simulink model "Energy_Cost03_04_2012"  (Simulink 7.5)
settings: Solver=ode45  StartTime=0.0  StopTime=24  RelTol=1e-3
model workspace: external: MAT-File (data not in the file)
libraries: simulink x4
(part 2 of 2)

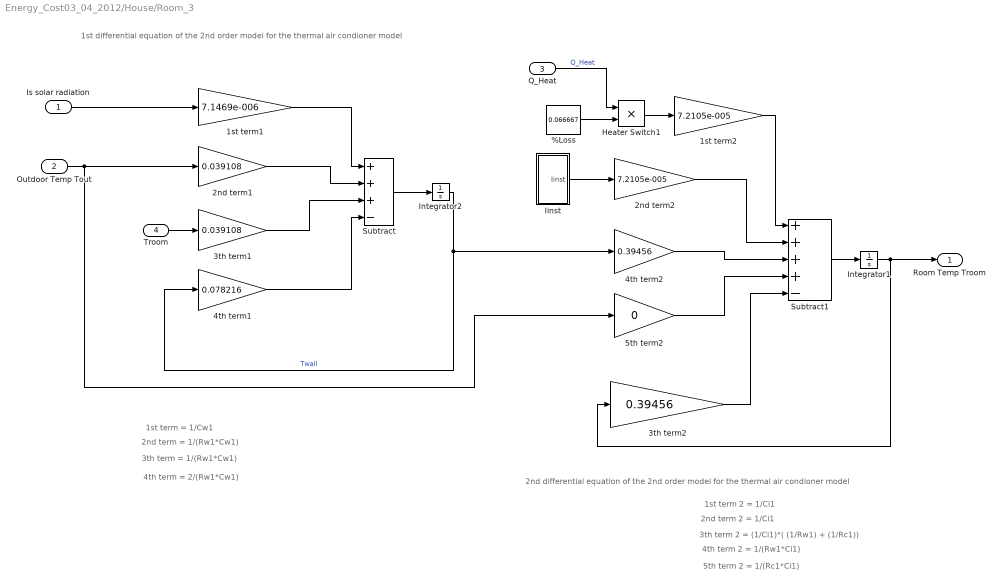
== system Energy_Cost03_04_2012/House/Room_3 ==
  note: 1st differential equation of the 2nd order
      | model for the thermal air condioner model
  note: 2nd differential equation of the 2nd order
      | model for the thermal air condioner model
  note: 1st term = 1/Cw1
  note: 2nd term = 1/(Rw1*Cw1)
  note: 3th term = 1/(Rw1*Cw1)
  note: 4th term = 2/(Rw1*Cw1)
  note: 1st term 2 = 1/Ci1
  note: 2nd term 2 = 1/Ci1
  note: 3th term 2 = (1/Ci1)*( (1/Rw1) + (1/Rc1))
  note: 4th term 2 = 1/(Rw1*Ci1)
  note: 5th term 2 = 1/(Rc1*Ci1)
  Is solar radiation : Inport
  Outdoor Temp Tout : Inport  Port=2
  Q_Heat : Inport  Port=3
  Troom : Inport  Port=4
  %Loss : Constant  Value=0.066667
  1st term1 : Gain  Gain=7.1469e-006
  1st term2 : Gain  Gain=7.2105e-005
  2nd term1 : Gain  Gain=0.039108
  2nd term2 : Gain  Gain=7.2105e-005
  3th term1 : Gain  Gain=0.039108
  3th term2 : Gain  Gain=0.39456
  4th term1 : Gain  Gain=0.078216
  4th term2 : Gain  Gain=0.39456
  5th term2 : Gain  Gain=0
  Heater Switch1 : Product  RndMeth=Zero
  Iinst : Subsystem
  Integrator1 : Integrator  InitialCondition=21
  Integrator2 : Integrator  InitialCondition=21
  Subtract : Sum  Inputs=+++-
  Subtract1 : Sum  Inputs=++++-
  Room Temp Troom : Outport  InitialOutput=0
  wires:
  2nd term1/1 -> Subtract/2
  4th term1/1 -> Subtract/4
  Subtract/1 -> Integrator2/1
  Integrator2/1 -> 4th term1/1, 4th term2/1  "Twall"
  Integrator1/1 -> 3th term2/1, Room Temp Troom/1
  Subtract1/1 -> Integrator1/1
  Outdoor Temp Tout/1 -> 2nd term1/1, 5th term2/1
  Troom/1 -> 3th term1/1
  3th term1/1 -> Subtract/3
  1st term1/1 -> Subtract/1
  2nd term2/1 -> Subtract1/2
  Q_Heat/1 -> Heater Switch1/1  "Q_Heat"
  Iinst/1(Iinst) -> 2nd term2/1
  Is solar radiation/1 -> 1st term1/1
  4th term2/1 -> Subtract1/3
  5th term2/1 -> Subtract1/4
  3th term2/1 -> Subtract1/5
  %Loss/1 -> Heater Switch1/2
  1st term2/1 -> Subtract1/1
  Heater Switch1/1 -> 1st term2/1

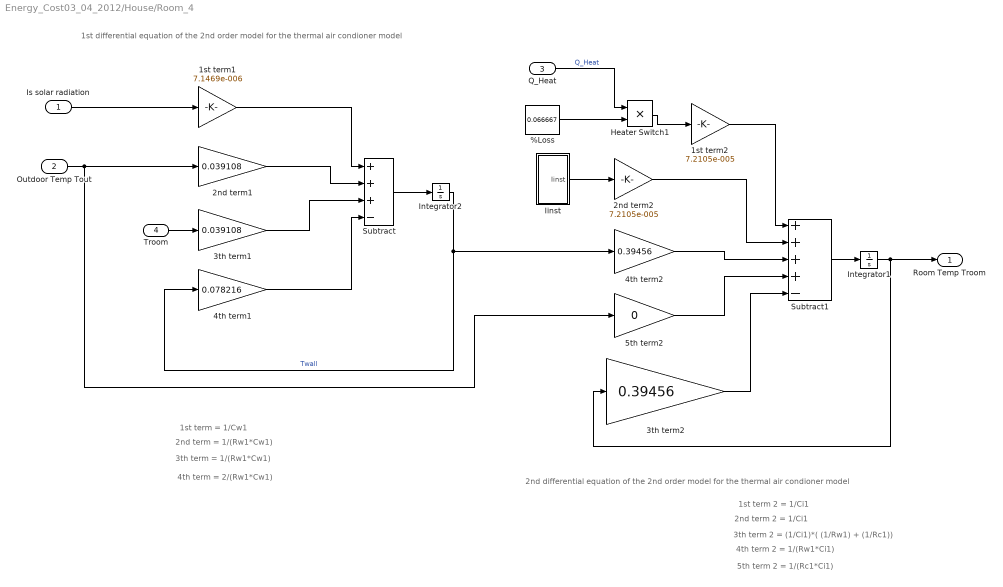
== system Energy_Cost03_04_2012/House/Room_4 ==
  note: 1st differential equation of the 2nd order
      | model for the thermal air condioner model
  note: 2nd differential equation of the 2nd order
      | model for the thermal air condioner model
  note: 1st term = 1/Cw1
  note: 2nd term = 1/(Rw1*Cw1)
  note: 3th term = 1/(Rw1*Cw1)
  note: 4th term = 2/(Rw1*Cw1)
  note: 1st term 2 = 1/Ci1
  note: 2nd term 2 = 1/Ci1
  note: 3th term 2 = (1/Ci1)*( (1/Rw1) + (1/Rc1))
  note: 4th term 2 = 1/(Rw1*Ci1)
  note: 5th term 2 = 1/(Rc1*Ci1)
  Is solar radiation : Inport
  Outdoor Temp Tout : Inport  Port=2
  Q_Heat : Inport  Port=3
  Troom : Inport  Port=4
  %Loss : Constant  Value=0.066667
  1st term1 : Gain  Gain=7.1469e-006
  1st term2 : Gain  Gain=7.2105e-005
  2nd term1 : Gain  Gain=0.039108
  2nd term2 : Gain  Gain=7.2105e-005
  3th term1 : Gain  Gain=0.039108
  3th term2 : Gain  Gain=0.39456
  4th term1 : Gain  Gain=0.078216
  4th term2 : Gain  Gain=0.39456
  5th term2 : Gain  Gain=0
  Heater Switch1 : Product  RndMeth=Zero
  Iinst : Subsystem
  Integrator1 : Integrator  InitialCondition=21
  Integrator2 : Integrator  InitialCondition=21
  Subtract : Sum  Inputs=+++-
  Subtract1 : Sum  Inputs=++++-
  Room Temp Troom : Outport  InitialOutput=0
  wires:
  2nd term1/1 -> Subtract/2
  4th term1/1 -> Subtract/4
  Subtract/1 -> Integrator2/1
  Integrator2/1 -> 4th term1/1, 4th term2/1  "Twall"
  Integrator1/1 -> 3th term2/1, Room Temp Troom/1
  Subtract1/1 -> Integrator1/1
  Outdoor Temp Tout/1 -> 2nd term1/1, 5th term2/1
  Troom/1 -> 3th term1/1
  3th term1/1 -> Subtract/3
  1st term1/1 -> Subtract/1
  2nd term2/1 -> Subtract1/2
  Q_Heat/1 -> Heater Switch1/1  "Q_Heat"
  Iinst/1(Iinst) -> 2nd term2/1
  Is solar radiation/1 -> 1st term1/1
  4th term2/1 -> Subtract1/3
  5th term2/1 -> Subtract1/4
  3th term2/1 -> Subtract1/5
  %Loss/1 -> Heater Switch1/2
  Heater Switch1/1 -> 1st term2/1
  1st term2/1 -> Subtract1/1

== system Energy_Cost03_04_2012/Lighting/Cost ==
  Powe_cons : Inport
  Bus Creator2 : BusCreator  Inputs=3
  Integrator : Integrator
  Integrator3 : Integrator
  PlotResults4 : Scope  NumInputPorts=2
      settings: TimeRange=24  YMin=0.027455~0.323  YMax=0.030345~0.357  SaveName=a18  DataFormat=Array
  Rates : Subsystem
      mask Display: % image(imread('Elec_stove.jpg'))
  To File : ToFile  Filename=Lighting_Total_LG  MatrixName=Detail_kWhr_Coshr_LG
  Watts-->kW : Gain  Gain=1/1000  SaturateOnIntegerOverflow=on  OutDataTypeStr=Inherit: Same as input  ParamDataTypeStr=Inherit: Same as input
  wires:
  Rates/1(Rate) -> Integrator/1
  Watts-->kW/1 -> Rates/1(Powe_cons), Integrator3/1, Bus Creator2/1
  Integrator3/1 -> PlotResults4/2, Bus Creator2/2  "kw_hr"
  Bus Creator2/1 -> To File/1
  Integrator/1 -> PlotResults4/1, Bus Creator2/3  "Cost_hr"
  Powe_cons/1 -> Watts-->kW/1

== system Energy_Cost03_04_2012/Lighting/Cost_CFL ==
  Powe_cons : Inport
  Bus Creator2 : BusCreator  Inputs=2
  Integrator1 : Integrator
  Integrator3 : Integrator
  PlotResults4 : Scope  NumInputPorts=2
      settings: TimeRange=24  YMin=0~0  YMax=0.018~0.21  SaveName=a18  DataFormat=Array
  Rates : Subsystem
      mask Display: % image(imread('Elec_stove.jpg'))
  To File3 : ToFile  Filename=CFL_LG  MatrixName=kW_Cos_CFL_LG
  Watts-->kW : Gain  Gain=1/1000  SaturateOnIntegerOverflow=on  OutDataTypeStr=Inherit: Same as input  ParamDataTypeStr=Inherit: Same as input
  wires:
  Rates/1(Rate) -> Integrator1/1
  Watts-->kW/1 -> Integrator3/1, Rates/1(Powe_cons)
  Integrator3/1 -> PlotResults4/2, Bus Creator2/1  "kw_hr"
  Powe_cons/1 -> Watts-->kW/1
  Integrator1/1 -> Bus Creator2/2, PlotResults4/1
  Bus Creator2/1 -> To File3/1

== system Energy_Cost03_04_2012/Lighting/Cost_FLU ==
  Powe_cons : Inport
  Bus Creator2 : BusCreator  Inputs=2
  Integrator : Integrator
  Integrator3 : Integrator
  PlotResults4 : Scope  NumInputPorts=2
      settings: TimeRange=24  YMin=0~0  YMax=0.018~0.21  SaveName=a18  DataFormat=Array
  Rates : Subsystem
      mask Display: % image(imread('Elec_stove.jpg'))
  To File4 : ToFile  Filename=CFLTubes_LG  MatrixName=kW_Cos_CFLTubes_LG
  Watts-->kW : Gain  Gain=1/1000  SaturateOnIntegerOverflow=on  OutDataTypeStr=Inherit: Same as input  ParamDataTypeStr=Inherit: Same as input
  wires:
  Rates/1(Rate) -> Integrator/1
  Watts-->kW/1 -> Integrator3/1, Rates/1(Powe_cons)
  Integrator3/1 -> PlotResults4/2, Bus Creator2/1  "kw_hr"
  Bus Creator2/1 -> To File4/1
  Integrator/1 -> PlotResults4/1, Bus Creator2/2  "Cost_hr"
  Powe_cons/1 -> Watts-->kW/1

== system Energy_Cost03_04_2012/Lighting/Cost_Inc ==
  Powe_cons : Inport
  Bus Creator2 : BusCreator  Inputs=2
  Integrator : Integrator
  Integrator3 : Integrator
  PlotResults4 : Scope  NumInputPorts=2
      settings: TimeRange=24  YMin=0~0  YMax=0.018~0.21  SaveName=a18  DataFormat=Array
  Rates : Subsystem
      mask Display: % image(imread('Elec_stove.jpg'))
  To File1 : ToFile  Filename=Inc_LG  MatrixName=kW_Cos_Inc_LG
  Watts-->kW : Gain  Gain=1/1000  SaturateOnIntegerOverflow=on  OutDataTypeStr=Inherit: Same as input  ParamDataTypeStr=Inherit: Same as input
  wires:
  Rates/1(Rate) -> Integrator/1
  Watts-->kW/1 -> Integrator3/1, Rates/1(Powe_cons)
  Integrator3/1 -> PlotResults4/2, Bus Creator2/1  "kw_hr"
  Bus Creator2/1 -> To File1/1
  Integrator/1 -> PlotResults4/1, Bus Creator2/2  "Cost_hr"
  Powe_cons/1 -> Watts-->kW/1

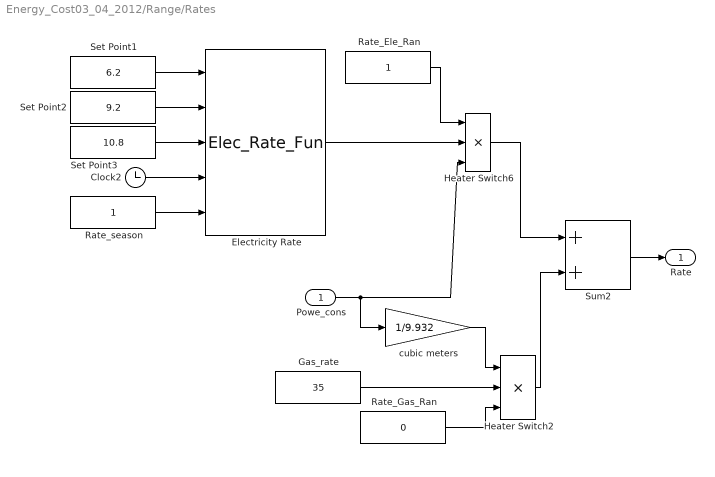
== system Energy_Cost03_04_2012/Range/Rates ==
  Powe_cons : Inport
  Clock2 : Clock
      settings: Decimation=100
  Electricity Rate : M-S-Function  FunctionName=Elec_Rate_Fun
      mask Display: fprintf('Elec_Rate_Fun %d',[] )
  Gas_rate : Constant  Value=35
  Heater Switch2 : Product  Inputs=3  RndMeth=Zero
  Heater Switch6 : Product  Inputs=3  RndMeth=Zero
  Rate_Ele_Ran : Constant
  Rate_Gas_Ran : Constant  Value=0
  Rate_season : Constant
  Set Point1 : Constant  Value=6.2
  Set Point2 : Constant  Value=9.2
  Set Point3 : Constant  Value=10.8
  Sum2 : Sum  SaturateOnIntegerOverflow=on  InputSameDT=on  OutDataTypeStr=Inherit: Same as first input
  cubic meters : Gain  Gain=1/9.932  SaturateOnIntegerOverflow=on  OutDataTypeStr=Inherit: Same as input  ParamDataTypeStr=Inherit: Same as input
  Rate : Outport  InitialOutput=0
  wires:
  Set Point1/1 -> Electricity Rate/1
  Set Point2/1 -> Electricity Rate/2
  Set Point3/1 -> Electricity Rate/3
  Clock2/1 -> Electricity Rate/4
  Electricity Rate/1 -> Heater Switch6/2
  Rate_season/1 -> Electricity Rate/5
  Rate_Ele_Ran/1 -> Heater Switch6/1
  Powe_cons/1 -> cubic meters/1, Heater Switch6/3
  cubic meters/1 -> Heater Switch2/1
  Gas_rate/1 -> Heater Switch2/2
  Rate_Gas_Ran/1 -> Heater Switch2/3
  Heater Switch6/1 -> Sum2/1
  Heater Switch2/1 -> Sum2/2
  Sum2/1 -> Rate/1

== system Energy_Cost03_04_2012/Refrigerator/Food ==
  Constant4 : Constant  Value=400
  Food : Outport  InitialOutput=0
  wires:
  Constant4/1 -> Food/1

== system Energy_Cost03_04_2012/Refrigerator/Rates ==
  Powe_cons : Inport
  Clock2 : Clock
      settings: Decimation=100
  Ele_mid : Constant  Value=9.2
  Ele_off : Constant  Value=6.2
  Ele_peak : Constant  Value=10.8
  Electricity Rate : M-S-Function  FunctionName=Elec_Rate_Fun
      mask Display: fprintf('Elec_Rate_Fun %d',[] )
  Gas rate : Constant  Value=35.7
  Heater Switch2 : Product  Inputs=3  RndMeth=Zero
  Heater Switch6 : Product  Inputs=3  RndMeth=Zero
  Rate_Ele_WH : Constant
  Rate_Gas_WH : Constant  Value=0
  Rate_season : Constant
  Sum2 : Sum  SaturateOnIntegerOverflow=on  InputSameDT=on  OutDataTypeStr=Inherit: Same as first input
  c3=Watts/Pc : Gain  Gain=1/9.932  SaturateOnIntegerOverflow=on  OutDataTypeStr=Inherit: Same as input  ParamDataTypeStr=Inherit: Same as input
  Rate : Outport  InitialOutput=0
  wires:
  Ele_off/1 -> Electricity Rate/1
  Ele_mid/1 -> Electricity Rate/2
  Ele_peak/1 -> Electricity Rate/3
  Clock2/1 -> Electricity Rate/4
  Electricity Rate/1 -> Heater Switch6/2
  Rate_season/1 -> Electricity Rate/5
  Rate_Ele_WH/1 -> Heater Switch6/1
  Powe_cons/1 -> c3=Watts/Pc/1, Heater Switch6/3
  c3=Watts/Pc/1 -> Heater Switch2/1
  Gas rate/1 -> Heater Switch2/2
  Rate_Gas_WH/1 -> Heater Switch2/3
  Heater Switch6/1 -> Sum2/1
  Heater Switch2/1 -> Sum2/2
  Sum2/1 -> Rate/1

== system Energy_Cost03_04_2012/Thermostat/If Action Subsystem ==
  In1 : Inport
  Action Port : ActionPort  ActionType=then
  Out1 : Outport
  wires:
  In1/1 -> Out1/1

== system Energy_Cost03_04_2012/Thermostat/If Action Subsystem1 ==
  In1 : Inport
  Action Port : ActionPort  ActionType=else
  Out1 : Outport
  wires:
  In1/1 -> Out1/1

== system Energy_Cost03_04_2012/Thermostat1/If Action Subsystem ==
  In1 : Inport
  Action Port : ActionPort  ActionType=then
  Out1 : Outport
  wires:
  In1/1 -> Out1/1

== system Energy_Cost03_04_2012/Thermostat1/If Action Subsystem1 ==
  In1 : Inport
  Action Port : ActionPort  ActionType=else
  Out1 : Outport
  wires:
  In1/1 -> Out1/1

== system Energy_Cost03_04_2012/Water Heater/Rates ==
  Powe_cons : Inport
  Clock2 : Clock
      settings: Decimation=100
  Ele_mid : Constant  Value=9.2
  Ele_off : Constant  Value=6.2
  Ele_peak : Constant  Value=10.8
  Electricity Rate : M-S-Function  FunctionName=Elec_Rate_Fun
      mask Display: fprintf('Elec_Rate_Fun %d',[] )
  Gas rate : Constant  Value=35.7
  Heater Switch2 : Product  Inputs=3  RndMeth=Zero
  Heater Switch6 : Product  Inputs=3  RndMeth=Zero
  Rate_Ele_WH : Constant  Value=0
  Rate_Gas_WH : Constant
  Rate_season : Constant
  Sum2 : Sum  SaturateOnIntegerOverflow=on  InputSameDT=on  OutDataTypeStr=Inherit: Same as first input
  c3=Watts/Pc : Gain  Gain=1/9.932  SaturateOnIntegerOverflow=on  OutDataTypeStr=Inherit: Same as input  ParamDataTypeStr=Inherit: Same as input
  Rate : Outport  InitialOutput=0
  wires:
  Ele_off/1 -> Electricity Rate/1
  Ele_mid/1 -> Electricity Rate/2
  Ele_peak/1 -> Electricity Rate/3
  Clock2/1 -> Electricity Rate/4
  Electricity Rate/1 -> Heater Switch6/2
  Rate_season/1 -> Electricity Rate/5
  Rate_Ele_WH/1 -> Heater Switch6/1
  Powe_cons/1 -> c3=Watts/Pc/1, Heater Switch6/3
  c3=Watts/Pc/1 -> Heater Switch2/1
  Gas rate/1 -> Heater Switch2/2
  Rate_Gas_WH/1 -> Heater Switch2/3
  Heater Switch6/1 -> Sum2/1
  Heater Switch2/1 -> Sum2/2
  Sum2/1 -> Rate/1

== system Energy_Cost03_04_2012/Air Conditioner/Cost_AA/Rates ==
  Powe_cons : Inport
  Clock1 : Clock
      settings: Decimation=100
  Constant : Constant  Value=6.2
  Constant1 : Constant  Value=9.2
  Constant2 : Constant  Value=10.8
  Constant3 : Constant
  Electricity Rate : M-S-Function  FunctionName=Elec_Rate_Fun
      mask Display: fprintf('Elec_Rate_Fun %d',[] )
  Heater Switch1 : Product  RndMeth=Zero
  Rate : Outport  InitialOutput=0
  wires:
  Constant/1 -> Electricity Rate/1
  Constant1/1 -> Electricity Rate/2
  Constant2/1 -> Electricity Rate/3
  Clock1/1 -> Electricity Rate/4
  Constant3/1 -> Electricity Rate/5
  Electricity Rate/1 -> Heater Switch1/1  "Elec_Rate"
  Powe_cons/1 -> Heater Switch1/2
  Heater Switch1/1 -> Rate/1

== system Energy_Cost03_04_2012/Furnace/Cost_FC/Rates ==
  Powe_cons : Inport
  Clock1 : Clock
      settings: Decimation=100
  Constant : Constant  Value=6.2
  Constant1 : Constant  Value=9.2
  Constant2 : Constant  Value=10.8
  Constant3 : Constant
  Electricity Rate : M-S-Function  FunctionName=Elec_Rate_Fun
      mask Display: fprintf('Elec_Rate_Fun %d',[] )
  Heater Switch1 : Product  RndMeth=Zero
  Rate : Outport  InitialOutput=0
  wires:
  Heater Switch1/1 -> Rate/1
  Powe_cons/1 -> Heater Switch1/2
  Electricity Rate/1 -> Heater Switch1/1  "Elec_Rate"
  Constant3/1 -> Electricity Rate/5
  Clock1/1 -> Electricity Rate/4
  Constant2/1 -> Electricity Rate/3
  Constant1/1 -> Electricity Rate/2
  Constant/1 -> Electricity Rate/1

== system Energy_Cost03_04_2012/House/Room_1/Iinst ==
  Constant : Constant  Value=20
  Constant1 : Constant  Value=5
  Constant2 : Constant  Value=-1
  Constant3 : Constant  Value=600
  Constant4 : Constant  Value=200
  Digital Clock : DigitalClock
  Divide : Product  Inputs=*/
  Heater Switch1 : Product  RndMeth=Zero
  Heater Switch2 : Product  RndMeth=Zero
  Heater Switch3 : Product  RndMeth=Zero
  Math Function1 : Math  SaturateOnIntegerOverflow=on
  Solar : Scope
      settings: TimeRange=50  YMin=0  YMax=40  SaveName=a6  DataFormat=Array
  Subtract1 : Sum
  Subtract2 : Sum  Inputs=+-
  Iinst : Outport  InitialOutput=0
  wires:
  Digital Clock/1 -> Subtract2/1
  Constant/1 -> Subtract2/2
  Subtract2/1 -> Heater Switch1/1, Heater Switch1/2
  Heater Switch1/1 -> Divide/1
  Constant1/1 -> Divide/2
  Divide/1 -> Heater Switch2/2
  Constant2/1 -> Heater Switch2/1
  Heater Switch2/1 -> Math Function1/1
  Math Function1/1 -> Heater Switch3/2
  Constant3/1 -> Heater Switch3/1
  Subtract1/1 -> Iinst/1, Solar/1
  Constant4/1 -> Subtract1/1
  Heater Switch3/1 -> Subtract1/2

== system Energy_Cost03_04_2012/House/Room_2/Iinst ==
  Clock : Clock
      settings: Decimation=10
  Constant : Constant  Value=20
  Constant1 : Constant  Value=5
  Constant2 : Constant  Value=-1
  Constant3 : Constant  Value=600
  Constant4 : Constant  Value=200
  Divide : Product  Inputs=*/
  Heater Switch1 : Product  RndMeth=Zero
  Heater Switch2 : Product  RndMeth=Zero
  Heater Switch3 : Product  RndMeth=Zero
  Math Function1 : Math  SaturateOnIntegerOverflow=on
  Solar : Scope
      settings: TimeRange=50  YMin=0  YMax=40  SaveName=a6  DataFormat=Array
  Subtract1 : Sum
  Subtract2 : Sum  Inputs=+-
  Iinst : Outport  InitialOutput=0
  wires:
  Clock/1 -> Subtract2/1
  Constant/1 -> Subtract2/2
  Subtract2/1 -> Heater Switch1/1, Heater Switch1/2
  Heater Switch1/1 -> Divide/1
  Constant1/1 -> Divide/2
  Divide/1 -> Heater Switch2/2
  Constant2/1 -> Heater Switch2/1
  Heater Switch2/1 -> Math Function1/1
  Math Function1/1 -> Heater Switch3/2
  Constant3/1 -> Heater Switch3/1
  Subtract1/1 -> Iinst/1, Solar/1
  Constant4/1 -> Subtract1/1
  Heater Switch3/1 -> Subtract1/2

== system Energy_Cost03_04_2012/House/Room_3/Iinst ==
  Clock : Clock
      settings: Decimation=10
  Constant : Constant  Value=20
  Constant1 : Constant  Value=5
  Constant2 : Constant  Value=-1
  Constant3 : Constant  Value=600
  Constant4 : Constant  Value=200
  Divide : Product  Inputs=*/
  Heater Switch1 : Product  RndMeth=Zero
  Heater Switch2 : Product  RndMeth=Zero
  Heater Switch3 : Product  RndMeth=Zero
  Math Function1 : Math  SaturateOnIntegerOverflow=on
  Solar : Scope
      settings: TimeRange=50  YMin=0  YMax=40  SaveName=a6  DataFormat=Array
  Subtract1 : Sum
  Subtract2 : Sum  Inputs=+-
  Iinst : Outport  InitialOutput=0
  wires:
  Clock/1 -> Subtract2/1
  Constant/1 -> Subtract2/2
  Subtract2/1 -> Heater Switch1/1, Heater Switch1/2
  Heater Switch1/1 -> Divide/1
  Constant1/1 -> Divide/2
  Divide/1 -> Heater Switch2/2
  Constant2/1 -> Heater Switch2/1
  Heater Switch2/1 -> Math Function1/1
  Math Function1/1 -> Heater Switch3/2
  Constant3/1 -> Heater Switch3/1
  Subtract1/1 -> Iinst/1, Solar/1
  Constant4/1 -> Subtract1/1
  Heater Switch3/1 -> Subtract1/2

== system Energy_Cost03_04_2012/House/Room_4/Iinst ==
  Clock : Clock
      settings: Decimation=10
  Constant : Constant  Value=20
  Constant1 : Constant  Value=5
  Constant2 : Constant  Value=-1
  Constant3 : Constant  Value=600
  Constant4 : Constant  Value=200
  Divide : Product  Inputs=*/
  Heater Switch1 : Product  RndMeth=Zero
  Heater Switch2 : Product  RndMeth=Zero
  Heater Switch3 : Product  RndMeth=Zero
  Math Function1 : Math  SaturateOnIntegerOverflow=on
  Solar : Scope
      settings: TimeRange=50  YMin=0  YMax=40  SaveName=a6  DataFormat=Array
  Subtract1 : Sum
  Subtract2 : Sum  Inputs=+-
  Iinst : Outport  InitialOutput=0
  wires:
  Clock/1 -> Subtract2/1
  Constant/1 -> Subtract2/2
  Subtract2/1 -> Heater Switch1/1, Heater Switch1/2
  Heater Switch1/1 -> Divide/1
  Constant1/1 -> Divide/2
  Divide/1 -> Heater Switch2/2
  Constant2/1 -> Heater Switch2/1
  Heater Switch2/1 -> Math Function1/1
  Math Function1/1 -> Heater Switch3/2
  Constant3/1 -> Heater Switch3/1
  Subtract1/1 -> Iinst/1, Solar/1
  Constant4/1 -> Subtract1/1
  Heater Switch3/1 -> Subtract1/2

== system Energy_Cost03_04_2012/Lighting/Cost/Rates ==
  Powe_cons : Inport
  Clock1 : Clock
      settings: Decimation=100
  Constant : Constant  Value=6.2
  Constant1 : Constant  Value=9.2
  Constant2 : Constant  Value=10.8
  Constant3 : Constant
  Electricity Rate : M-S-Function  FunctionName=Elec_Rate_Fun
      mask Display: fprintf('Elec_Rate_Fun %d',[] )
  Heater Switch1 : Product  RndMeth=Zero
  Rate : Outport  InitialOutput=0
  wires:
  Constant/1 -> Electricity Rate/1
  Constant1/1 -> Electricity Rate/2
  Constant2/1 -> Electricity Rate/3
  Clock1/1 -> Electricity Rate/4
  Constant3/1 -> Electricity Rate/5
  Electricity Rate/1 -> Heater Switch1/1  "Elec_Rate"
  Powe_cons/1 -> Heater Switch1/2
  Heater Switch1/1 -> Rate/1

== system Energy_Cost03_04_2012/Lighting/Cost_CFL/Rates ==
  Powe_cons : Inport
  Clock1 : Clock
      settings: Decimation=100
  Constant : Constant  Value=6.2
  Constant1 : Constant  Value=9.2
  Constant2 : Constant  Value=10.8
  Constant3 : Constant
  Electricity Rate : M-S-Function  FunctionName=Elec_Rate_Fun
      mask Display: fprintf('Elec_Rate_Fun %d',[] )
  Heater Switch1 : Product  RndMeth=Zero
  Rate : Outport  InitialOutput=0
  wires:
  Constant/1 -> Electricity Rate/1
  Constant1/1 -> Electricity Rate/2
  Constant2/1 -> Electricity Rate/3
  Clock1/1 -> Electricity Rate/4
  Constant3/1 -> Electricity Rate/5
  Electricity Rate/1 -> Heater Switch1/1  "Elec_Rate"
  Powe_cons/1 -> Heater Switch1/2
  Heater Switch1/1 -> Rate/1

== system Energy_Cost03_04_2012/Lighting/Cost_FLU/Rates ==
  Powe_cons : Inport
  Clock1 : Clock
      settings: Decimation=100
  Constant : Constant  Value=6.2
  Constant1 : Constant  Value=9.2
  Constant2 : Constant  Value=10.8
  Constant3 : Constant
  Electricity Rate : M-S-Function  FunctionName=Elec_Rate_Fun
      mask Display: fprintf('Elec_Rate_Fun %d',[] )
  Heater Switch1 : Product  RndMeth=Zero
  Rate : Outport  InitialOutput=0
  wires:
  Constant/1 -> Electricity Rate/1
  Constant1/1 -> Electricity Rate/2
  Constant2/1 -> Electricity Rate/3
  Clock1/1 -> Electricity Rate/4
  Constant3/1 -> Electricity Rate/5
  Electricity Rate/1 -> Heater Switch1/1  "Elec_Rate"
  Powe_cons/1 -> Heater Switch1/2
  Heater Switch1/1 -> Rate/1

== system Energy_Cost03_04_2012/Lighting/Cost_Inc/Rates ==
  Powe_cons : Inport
  Clock1 : Clock
      settings: Decimation=100
  Constant : Constant  Value=6.2
  Constant1 : Constant  Value=9.2
  Constant2 : Constant  Value=10.8
  Constant3 : Constant
  Electricity Rate1 : M-S-Function  FunctionName=Elec_Rate_Fun
      mask Display: fprintf('Elec_Rate_Fun %d',[] )
  Heater Switch1 : Product  RndMeth=Zero
  Rate : Outport  InitialOutput=0
  wires:
  Constant/1 -> Electricity Rate1/1
  Constant1/1 -> Electricity Rate1/2
  Constant2/1 -> Electricity Rate1/3
  Clock1/1 -> Electricity Rate1/4
  Constant3/1 -> Electricity Rate1/5
  Electricity Rate1/1 -> Heater Switch1/1  "Elec_Rate"
  Powe_cons/1 -> Heater Switch1/2
  Heater Switch1/1 -> Rate/1
